simulink model "integr_comp"  (R2022b)
settings: Solver=VariableStepAuto  StartTime=0.0  StopTime=0.01  RelTol=1e-3
settings Model: Creator=isaac  LastModifiedBy=isaac

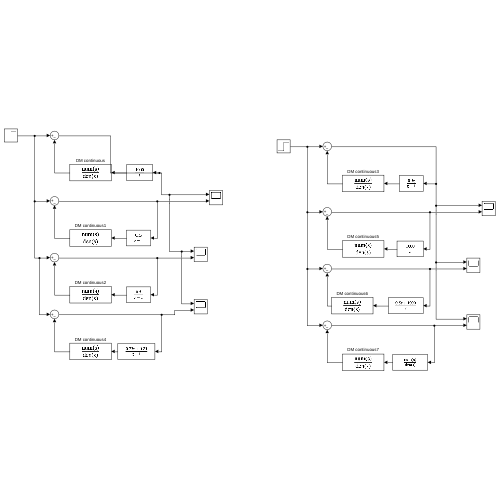
[thumbnail: Simulink's stored preview of the top-level diagram]
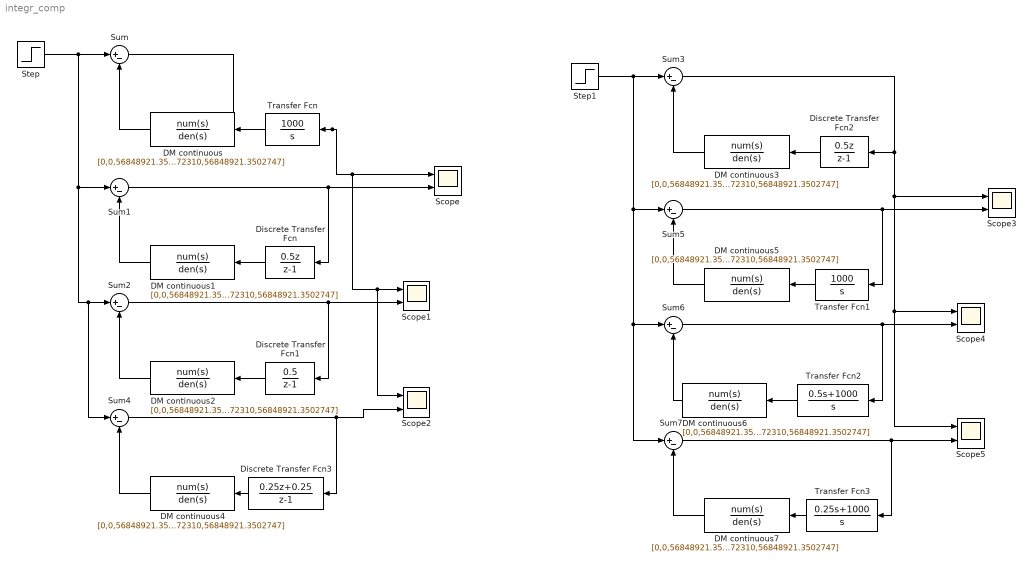
== system integr_comp ==
  DM continuous{,1..7} (8 alike) : TransferFcn  Numerator=[0,0,56848921.3502747]  Denominator=[1,1507.96447372310,56848921.3502747]
  Discrete Transfer Fcn : DiscreteTransferFcn  Numerator=[0.5 0]  Denominator=[1 -1]  SampleTime=0.0005
  Discrete Transfer Fcn1 : DiscreteTransferFcn  Numerator=[0.5]  Denominator=[1 -1]  SampleTime=0.0005
  Discrete Transfer Fcn2 : DiscreteTransferFcn  Numerator=[0.5 0]  Denominator=[1 -1]  SampleTime=0.0005
  Discrete Transfer Fcn3 : DiscreteTransferFcn  Numerator=[0.25 0.25]  Denominator=[1 -1]  SampleTime=0.0005
  Scope{,1..5} (6 alike) : Scope  NumInputPorts=2
  Step : Step  Before=1  SampleTime=0.0001
  Step1 : Step  Before=1  SampleTime=0.0001
  Sum{,1..7} (8 alike) : Sum  Inputs=|+-
  Transfer Fcn : TransferFcn  Numerator=[1000]  Denominator=[1 0]
  Transfer Fcn1 : TransferFcn  Numerator=[1000]  Denominator=[1 0]
  Transfer Fcn2 : TransferFcn  Numerator=[0.5 1000]  Denominator=[1 0]
  Transfer Fcn3 : TransferFcn  Numerator=[0.25 1000]  Denominator=[1 0]
  wires:
  DM continuous/1 -> Sum/2
  Sum/1 -> Transfer Fcn/1, Scope2/1, Scope1/1, Scope/1
  Transfer Fcn/1 -> DM continuous/1
  DM continuous1/1 -> Sum1/2
  Discrete Transfer Fcn/1 -> DM continuous1/1
  Sum1/1 -> Discrete Transfer Fcn/1, Scope/2
  Sum2/1 -> Scope1/2, Discrete Transfer Fcn1/1
  Discrete Transfer Fcn1/1 -> DM continuous2/1
  DM continuous2/1 -> Sum2/2
  Sum4/1 -> Scope2/2, Discrete Transfer Fcn3/1
  Discrete Transfer Fcn3/1 -> DM continuous4/1
  Step/1 -> Sum1/1, Sum4/1, Sum2/1, Sum/1
  DM continuous4/1 -> Sum4/2
  DM continuous3/1 -> Sum3/2
  DM continuous7/1 -> Sum7/2
  Sum5/1 -> Transfer Fcn1/1, Scope3/2
  Sum3/1 -> Discrete Transfer Fcn2/1, Scope4/1, Scope5/1, Scope3/1
  Step1/1 -> Sum5/1, Sum7/1, Sum6/1, Sum3/1
  Transfer Fcn3/1 -> DM continuous7/1
  Sum7/1 -> Transfer Fcn3/1, Scope5/2
  Transfer Fcn2/1 -> DM continuous6/1
  DM continuous5/1 -> Sum5/2
  DM continuous6/1 -> Sum6/2
  Sum6/1 -> Transfer Fcn2/1, Scope4/2
  Transfer Fcn1/1 -> DM continuous5/1
  Discrete Transfer Fcn2/1 -> DM continuous3/1
